simulink model "lab3_teil2fcn"  (R2018b)
settings: Solver=ode23t  StartTime=0.0  StopTime=10.0  RelTol=1e-12  AbsTol=1e-12
values from neighbouring files (symbols this model uses):
  AB = n * pi/4 * dB^2    (= 4.31026512073e-05)    [lab3_teil2.m]    (also in lab3_teil3.m; modelbildung_lab3.m)
  AK = pi/4 * dK^2    (= 0.000314159265359)    [lab3_teil2.m]    (also in lab3_teil3.m; modelbildung_lab3.m)
  FR = 5    [lab3_teil2.m]    (also in lab3_teil3.m; modelbildung_lab3.m)
  KI = 0.0005    [lab3_teil2.m]
  m = 1    [lab3_teil2.m]    (also in lab3_teil3.m; modelbildung_lab3.m)
  rho = 850    [lab3_teil2.m]    (also in lab3_teil3.m; modelbildung_lab3.m)
  xdotdot_soll = -100    [lab3_teil2.m]
  zeta = 0.5    [lab3_teil2.m]    (also in lab3_teil3.m; modelbildung_lab3.m)
libraries: simulink x1
settings Model: Creator=Naveen  LastModifiedBy=Naveen

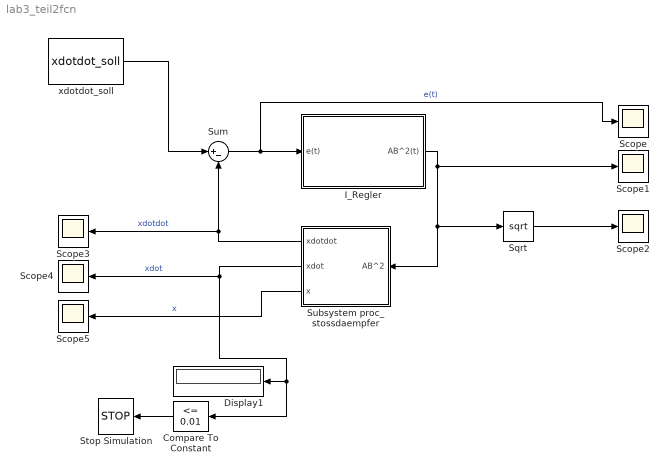
== system lab3_teil2fcn ==
  Compare To Constant : simulink/Logic and Bit Operations/Compare To Constant  relop=<=  const=0.01  OutDataTypeStr=boolean
  Display1 : Display
  I_Regler : Subsystem
  Scope{,1..5} (6 alike) : Scope
  Sqrt : Sqrt  SaturateOnIntegerOverflow=on
  Stop Simulation : Stop
  Subsystem proc_stossdaempfer : Subsystem
  Sum : Sum  Inputs=|+-
  xdotdot_soll : Constant  Value=xdotdot_soll
  wires:
  Compare To Constant/1 -> Stop Simulation/1
  Subsystem proc_stossdaempfer/3(x) -> Scope5/1  "x"
  Subsystem proc_stossdaempfer/2(xdot) -> Scope4/1, Compare To Constant/1, Display1/1  "xdot"
  Subsystem proc_stossdaempfer/1(xdotdot) -> Scope3/1, Sum/2  "xdotdot"
  xdotdot_soll/1 -> Sum/1
  Sum/1 -> Scope/1, I_Regler/1(e(t))  "e(t)"
  I_Regler/1(AB^2(t)) -> Scope1/1, Sqrt/1, Subsystem proc_stossdaempfer/1(AB^2)
  Sqrt/1 -> Scope2/1

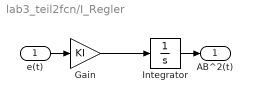
== system lab3_teil2fcn/I_Regler ==
  e(t) : Inport
  Gain : Gain  Gain=KI
  Integrator : Integrator  InitialCondition=AB^2  LimitOutput=on  LowerSaturationLimit=AB^2/1000
  AB^2(t) : Outport
  wires:
  e(t)/1 -> Gain/1
  Integrator/1 -> AB^2(t)/1
  Gain/1 -> Integrator/1

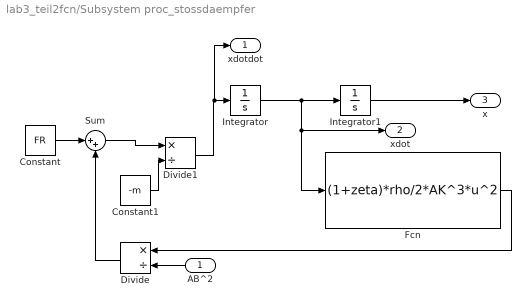
== system lab3_teil2fcn/Subsystem proc_stossdaempfer ==
  AB^2 : Inport
  Constant : Constant  Value=FR
  Constant1 : Constant  Value=-m
  Divide : Product  Inputs=*/
  Divide1 : Product  Inputs=*/
  Fcn : Fcn  Expr=(1+zeta)*rho/2*AK^3*u^2
  Integrator : Integrator  InitialCondition=3
  Integrator1 : Integrator  LimitOutput=on  LowerSaturationLimit=0
  Sum : Sum  Inputs=|++
  xdotdot : Outport
  xdot : Outport  Port=2
  x : Outport  Port=3
  wires:
  AB^2/1 -> Divide/2
  Integrator1/1 -> x/1
  Sum/1 -> Divide1/1
  Fcn/1 -> Divide/1
  Divide1/1 -> Integrator/1, xdotdot/1
  Constant/1 -> Sum/1
  Constant1/1 -> Divide1/2
  Divide/1 -> Sum/2
  Integrator/1 -> Integrator1/1, xdot/1, Fcn/1
